simulink model "Fig528"  (R2014b)
settings: Solver=ode3  StartTime=0.0  StopTime=10.001  FixedStep=2e-7  RelTol=1e-5
libraries: commutil2 x3, commanapbnd3 x3, commseqgen2 x3, powerlib_meascontrol x3, commfilt2 x1, commsink2 x1, commrandsrc2 x1
settings Model: Creator=Dennis Silage  LastModifiedBy=Silage
settings DataIOCC: SignalLoggingSaveFormat=ModelDataLogs
settings OptimizationCC: ExpressionDepthLimit=2147483647  InitFltsAndDblsToZero=on
settings DebuggingCC: UnderspecifiedInitializationDetection=Classic  MergeDetectMultiDrivingBlocksExec=none  SolverPrmCheckMsg=none  FcnCallInpInsideContextMsg=UseLocalSettings  StateNameClashWarn=warning
settings GRTTargetCC: CombineOutputUpdateFcns=off  GRTInterface=on

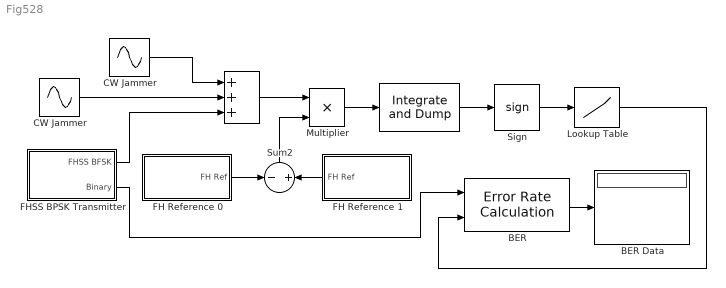
== system Fig528 ==
  " " : commfilt2/Integrate and Dump  obssamples=5000  offsetsamples=0  nodump=off  roundingMode=Floor  overflowMode=off
  "      " : Sum  Inputs=+++
  " CW Jammer " : Sin  Amplitude=25  Frequency=19400*pi  SampleTime=2e-7
  BER : commsink2/Error Rate Calculation  N=2  st_delay=0  cp_mode=Entire frame  subframe=[]  PMode=Port  WsName=ErrorVec  RsMode2=off  stop=off  numErr=100  maxBits=1e6
  BER Data : Display
  CW Jammer : Sin  Amplitude=25  Frequency=210000*pi  SampleTime=2e-7
  FH Reference 0 : Subsystem
  FH Reference 1 : Subsystem
  FHSS BPSK Transmitter : Subsystem
  Lookup Table : Lookup_n-D  NumberOfTableDimensions=1  BreakpointsForDimension1=[-1, 0, 1]  BreakpointsForDimension3=[5, 7]  Table=[0, 0, 1]  InternalRulePriority=Speed  RndMeth=Simplest  InputSameDT=on
  Multiplier : Product  RndMeth=Zero
  Sign : Signum
  Sum2 : Sum  Inputs=-+
  wires:
  Sign/1 -> Lookup Table/1
  BER/1 -> BER Data/1
  Multiplier/1 -> " "/1
  " "/1 -> Sign/1
  Sum2/1 -> Multiplier/2
  FH Reference 0/1(FH Ref) -> Sum2/1
  FH Reference 1/1(FH Ref) -> Sum2/2
  Lookup Table/1 -> BER/2
  FHSS BPSK Transmitter/2(Binary) -> BER/1
  "      "/1 -> Multiplier/1
  FHSS BPSK Transmitter/1(FHSS BFSK) -> "      "/3
  " CW Jammer "/1 -> "      "/2
  CW Jammer/1 -> "      "/1

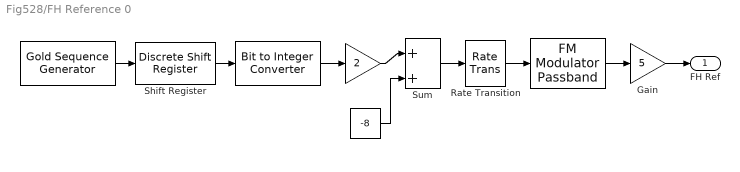
== system Fig528/FH Reference 0 ==
  "  " : commutil2/Bit to Integer Converter  nbits=3  bitOrder=MSB first  signedOutputValues=Unsigned  outDtype=Inherit via internal rule  outDtypeSigned=Inherit via internal rule
  "   " : Gain  Gain=2
  "    " : Constant  Value=-8
  "        " : commanapbnd3/FM Modulator Passband  Fc=100000  Ph=0  Kc=1000
  "           " : commseqgen2/Gold Sequence Generator  genPoly1=[1 0 0 1 0 1]  iniState1=[1 1 1 0 1]  genPoly2=[1 1 1 1 0 1]  iniState2=[1 0 0 0 1]  index=0  shift=0  outVarSiz=off  maxOutSizeMode=Dialog parameter  maxOutSize=[10 1]  ts=5e-5  frameBased=off  sampPerFrame=1  reset=off  outDataType=double
  Gain : Gain  Gain=5
  Rate Transition : RateTransition  OutPortSampleTime=2e-7
  Shift Register : powerlib_meascontrol/Additional Components/Discrete Shift Register  NSamples=3  InitialValue=0  Ts=5e-5
  Sum : Sum  Inputs=|++
  FH Ref : Outport
  wires:
  "   "/1 -> Sum/1
  Rate Transition/1 -> "        "/1
  Gain/1 -> FH Ref/1
  "  "/1 -> "   "/1
  "        "/1 -> Gain/1
  Sum/1 -> Rate Transition/1
  "           "/1 -> Shift Register/1
  "    "/1 -> Sum/2
  Shift Register/1 -> "  "/1

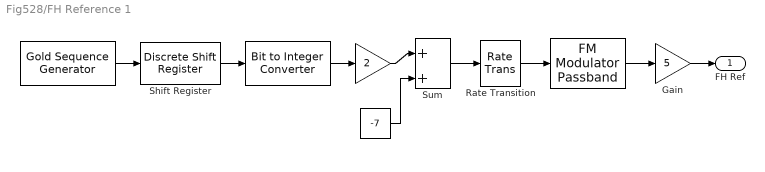
== system Fig528/FH Reference 1 ==
  "  " : commutil2/Bit to Integer Converter  nbits=3  bitOrder=MSB first  signedOutputValues=Unsigned  outDtype=Inherit via internal rule  outDtypeSigned=Inherit via internal rule
  "   " : Gain  Gain=2
  "    " : Constant  Value=-7
  "        " : commanapbnd3/FM Modulator Passband  Fc=100000  Ph=0  Kc=1000
  "           " : commseqgen2/Gold Sequence Generator  genPoly1=[1 0 0 1 0 1]  iniState1=[1 1 1 0 1]  genPoly2=[1 1 1 1 0 1]  iniState2=[1 0 0 0 1]  index=0  shift=0  outVarSiz=off  maxOutSizeMode=Dialog parameter  maxOutSize=[10 1]  ts=5e-5  frameBased=off  sampPerFrame=1  reset=off  outDataType=double
  Gain : Gain  Gain=5
  Rate Transition : RateTransition  OutPortSampleTime=2e-7
  Shift Register : powerlib_meascontrol/Additional Components/Discrete Shift Register  NSamples=3  InitialValue=0  Ts=5e-5
  Sum : Sum  Inputs=|++
  FH Ref : Outport
  wires:
  "   "/1 -> Sum/1
  Rate Transition/1 -> "        "/1
  Gain/1 -> FH Ref/1
  "  "/1 -> "   "/1
  "        "/1 -> Gain/1
  Sum/1 -> Rate Transition/1
  "           "/1 -> Shift Register/1
  "    "/1 -> Sum/2
  Shift Register/1 -> "  "/1

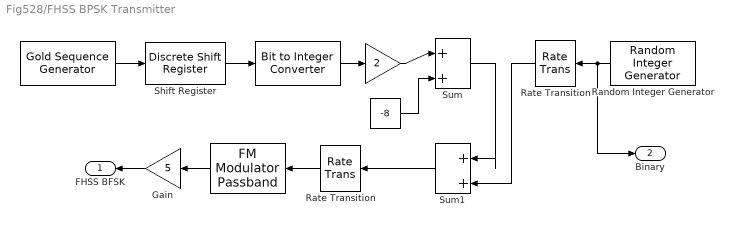
== system Fig528/FHSS BPSK Transmitter ==
  " " : commseqgen2/Gold Sequence Generator  genPoly1=[1 0 0 1 0 1]  iniState1=[1 1 1 0 1]  genPoly2=[1 1 1 1 0 1]  iniState2=[1 0 0 0 1]  index=0  shift=0  outVarSiz=off  maxOutSizeMode=Dialog parameter  maxOutSize=[10 1]  ts=5e-5  frameBased=off  sampPerFrame=1  reset=off  outDataType=double
  "  " : commutil2/Bit to Integer Converter  nbits=3  bitOrder=MSB first  signedOutputValues=Unsigned  outDtype=Inherit via internal rule  outDtypeSigned=Inherit via internal rule
  "   " : Gain  Gain=2
  "    " : Constant  Value=-8
  "        " : commanapbnd3/FM Modulator Passband  Fc=100000  Ph=0  Kc=1000
  Gain : Gain  Gain=5
  Random Integer Generator : commrandsrc2/Random Integer Generator  mul=2  seed=randseed  Ts=1e-3  frameBased=off  sampPerFrame=50  orient=on  outDataType=double
  Rate Transition : RateTransition  OutPortSampleTime=2e-7
  Rate Transition : RateTransition  OutPortSampleTime=5e-5
  Shift Register : powerlib_meascontrol/Additional Components/Discrete Shift Register  NSamples=3  InitialValue=0  Ts=5e-5
  Sum : Sum  Inputs=|++
  Sum1 : Sum  Inputs=|++
  FHSS BFSK : Outport
  Binary : Outport  Port=2
  wires:
  Random Integer Generator/1 -> Binary/1, Rate Transition/1
  "        "/1 -> Gain/1
  " "/1 -> Shift Register/1
  Shift Register/1 -> "  "/1
  "  "/1 -> "   "/1
  Sum1/1 -> Rate Transition/1
  Rate Transition/1 -> "        "/1
  Sum/1 -> Sum1/1
  Rate Transition/1 -> Sum1/2
  "    "/1 -> Sum/2
  "   "/1 -> Sum/1
  Gain/1 -> FHSS BFSK/1
